simulink model "vehicle_model_simulation_discrete"  (R2016a)
settings: Solver=FixedStepDiscrete  StartTime=0.0  StopTime=42  FixedStep=0.01  RelTol=1e-3
PostLoadFcn:
  | , if any(exist('dsrtsu_mdlpostloadfcn', 'file') == [2, 3, 6]), try dsrtsu_mdlpostloadfcn('Execute', bdroot); catch fprintf('Error in PostLoadFcn (dsrtsu_mdlpostloadfcn) for model "%s":\n %s\n', bdroot, lasterr); end, end,
values from neighbouring files (symbols this model uses):
  vx = 7/3.6    (= 1.94444444444)    [single_ctrl_est_design.m]
undefined symbols (not defined in the file or in its folder): DiscIntNeverNeededParam
libraries: simulink_extras x3, cstblocks x1
settings Model: DSRTSU_INTERNAL_RTI_VER=490  DSRTSU_INTERNAL_RTI_TYPE=rti1401  RTICANMMDATA=struct('GeneralSetupData',struct('modelroot','Z:\Workspace\Tools\Vehicle_Model\single_track_model','generalsettings',struct('filesettings',struct('destfolder',struct('Name','RTICANMM_FILES','Check',1),'buildfolder',struct('Name','.','Check',1),'AbsDestfolder',struct('Name','Z:\Workspace\Tools\Vehicle_Model\single_track_model\RTICANMM_FILES'),'AbsBuildfolder',struct('Name','Z:\Workspace\Tools\Vehicle_Model\single_track_model'))),'options',struct('addpaths',1,'rmpaths',1,'addtrcexclusion',logical(1),'cannavigator',struct('checkmonitoring',0),'show_usrtrc',0,'use_usrtrc',0),'advanced',struct('options',[1 1 1 1 1 1 1 1 1 1 1 1 1 1 1 1 1 1 1 1 1 1 1 1 1 1 1 1 1 1 1 1 1 1 1 1 1 1 1 1 1 1 1 1 1 1 1 1 1 1 1 1 1 1 1 1 1 1 1 1 1 1 1 1 1 1 1 1 1 1 1 1 1 1 1 1 1 1 1 1 1 1 1 1 1 1 1 1 1 1 1 1 1 1 1 1 1 1 1 1]),'MPSetup',{{}},'modelname','vehicle_model_simulation_discrete','block','vehicle_model_simulation_discrete'))  DSRTSU_INTERNAL_RTIFLEXRAYCONFIG=100  DSRTSU_INTERNAL_RTIFPGA=80  Creator=innovacion  LastModifiedBy=innovacion
settings OptimizationCC: BlockReduction=off  OptimizeBlockIOStorage=off  BufferReuse=off  GlobalBufferReuse=off  ExpressionFolding=off  LocalBlockOutputs=off
settings HardwareCC: ProdBitPerPointer=32  ProdLargestAtomicInteger=Integer  ProdEndianess=BigEndian  ProdWordSize=32  ProdHWDeviceType=Custom Processor->Custom  TargetIntDivRoundTo=Zero  TargetEndianess=BigEndian  TargetHWDeviceType=Custom Processor->Custom
settings RTWCC: SystemTargetFile=rti1401.tlc  MakeCommand=make_rti  TemplateMakefile=rti1401.tmf  Description=dSPACE DS1401 Hardware Platform
settings STFCustomTargetCC: ParMdlRefBuildCompliant=on  MatFileLogging=on  GRTInterface=off  SystemTargetFile=rti1401.tlc
settings GRTTargetCC: CompOptLevelCompliant=off  ConcurrentExecutionCompliant=off  GeneratePreprocessorConditionals=Use local settings  CombineOutputUpdateFcns=off  CPPClassGenCompliant=off  UseToolchainInfoCompliant=off

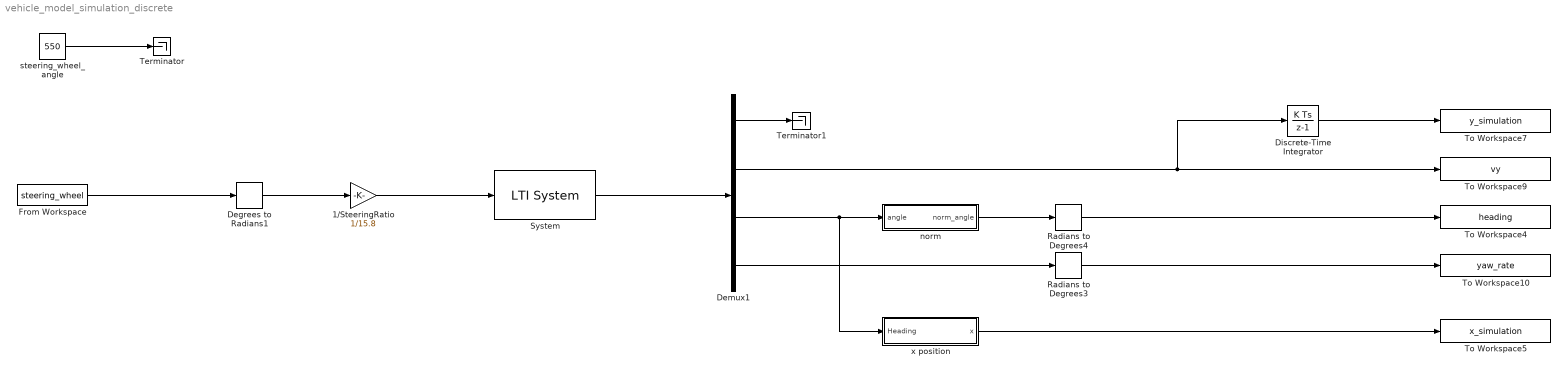
== system vehicle_model_simulation_discrete ==
  1/SteeringRatio : Gain  Gain=1/15.8
  Degrees to Radians1 : simulink_extras/Transformations/Degrees to Radians
  Demux1 : Demux
  Discrete-Time Integrator : DiscreteIntegrator  InitialConditionSetting=State (most efficient)  SampleTime=0.01  ICPrevOutput=DiscIntNeverNeededParam  ICPrevScaledInput=DiscIntNeverNeededParam
  From Workspace : FromWorkspace  VariableName=steering_wheel  SampleTime=0.01
  Radians to Degrees3 : simulink_extras/Transformations/Radians to Degrees
  Radians to Degrees4 : simulink_extras/Transformations/Radians to Degrees
  System : cstblocks/LTI System  sys=tf_systemd  IC=[]
  Terminator : Terminator
  Terminator1 : Terminator
  To Workspace10 : ToWorkspace  VariableName=yaw_rate  SaveFormat=Timeseries  SampleTime=-1
  To Workspace4 : ToWorkspace  VariableName=heading  SaveFormat=Timeseries  SampleTime=-1
  To Workspace5 : ToWorkspace  VariableName=x_simulation  SaveFormat=Timeseries  SampleTime=-1
  To Workspace7 : ToWorkspace  VariableName=y_simulation  SaveFormat=Timeseries  SampleTime=-1
  To Workspace9 : ToWorkspace  VariableName=vy  SaveFormat=Timeseries  SampleTime=-1
  norm : Subsystem
  steering_wheel_angle : Constant  Value=550  SampleTime=0.01
  x position : Subsystem
  wires:
  steering_wheel_angle/1 -> Terminator/1
  1/SteeringRatio/1 -> System/1
  Degrees to Radians1/1 -> 1/SteeringRatio/1
  System/1 -> Demux1/1
  Demux1/4 -> Radians to Degrees3/1
  Demux1/2 -> Discrete-Time Integrator/1, To Workspace9/1
  Demux1/3 -> norm/1(angle), x position/1(Heading)
  Radians to Degrees4/1 -> To Workspace4/1
  Radians to Degrees3/1 -> To Workspace10/1
  From Workspace/1 -> Degrees to Radians1/1
  norm/1(norm_angle) -> Radians to Degrees4/1
  Demux1/1 -> Terminator1/1
  x position/1(x) -> To Workspace5/1
  Discrete-Time Integrator/1 -> To Workspace7/1

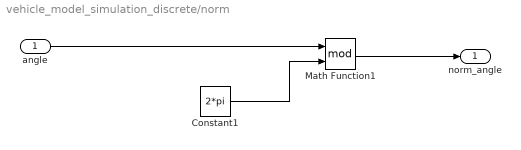
== system vehicle_model_simulation_discrete/norm ==
  angle : Inport
  Constant1 : Constant  Value=2*pi
  Math Function1 : Math  Operator=mod  OutputSignalType=real  SaturateOnIntegerOverflow=on
  norm_angle : Outport
  wires:
  Math Function1/1 -> norm_angle/1
  angle/1 -> Math Function1/1
  Constant1/1 -> Math Function1/2

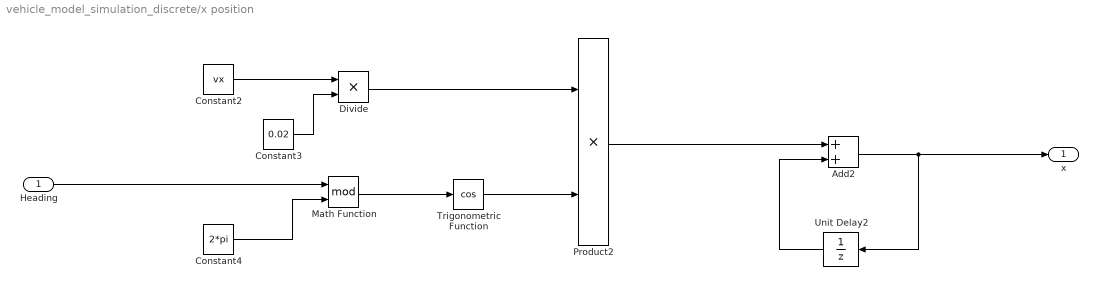
== system vehicle_model_simulation_discrete/x position ==
  Heading : Inport
  Add2 : Sum
  Constant2 : Constant  Value=vx
  Constant3 : Constant  Value=0.02
  Constant4 : Constant  Value=2*pi
  Divide : Product  Inputs=**
  Math Function : Math  Operator=mod  OutputSignalType=real  SaturateOnIntegerOverflow=on
  Product2 : Product
  Trigonometric Function : Trigonometry  Operator=cos
  Unit Delay2 : UnitDelay  SampleTime=-1
  x : Outport
  wires:
  Trigonometric Function/1 -> Product2/2
  Constant4/1 -> Math Function/2
  Math Function/1 -> Trigonometric Function/1
  Constant2/1 -> Divide/1
  Constant3/1 -> Divide/2
  Divide/1 -> Product2/1
  Unit Delay2/1 -> Add2/2
  Product2/1 -> Add2/1
  Add2/1 -> x/1, Unit Delay2/1
  Heading/1 -> Math Function/1
